simulink model "Model"  (R2023b)
settings: Solver=VariableStepAuto  StartTime=0.0  StopTime=10.0  RelTol=1e-3
values from neighbouring files (symbols this model uses):
  sys = System()    [Aflevering_3.m]
libraries: slpidlib x4
settings Model: Creator=JesperBertelsen  LastModifiedBy=JesperBertelsen

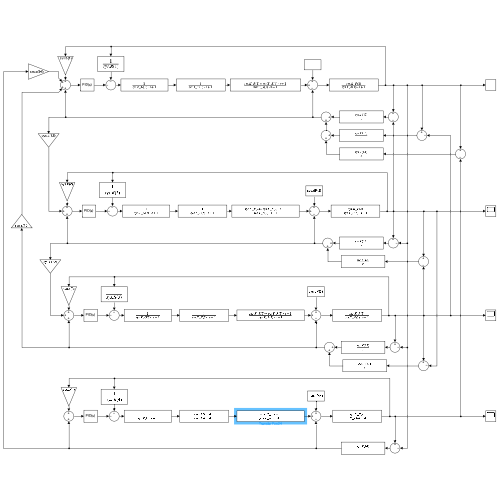
[thumbnail: Simulink's stored preview of the top-level diagram]
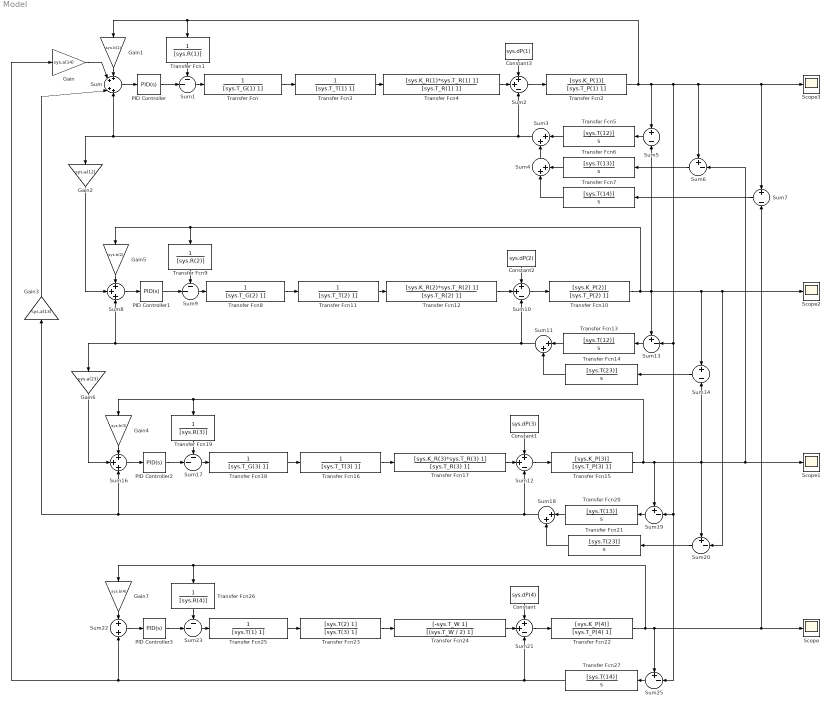
== system Model ==
  Constant : Constant  Value=sys.dP(4)
  Constant1 : Constant  Value=sys.dP(3)
  Constant2 : Constant  Value=sys.dP(2)
  Constant3 : Constant  Value=sys.dP(1)
  Gain : Gain  Gain=sys.a(14)
  Gain1 : Gain  Gain=sys.b(1)
  Gain2 : Gain  Gain=sys.a(12)
  Gain3 : Gain  Gain=sys.a(13)
  Gain4 : Gain  Gain=sys.b(3)
  Gain5 : Gain  Gain=sys.b(2)
  Gain6 : Gain  Gain=sys.a(23)
  Gain7 : Gain  Gain=sys.b(4)
  PID Controller{,1..3} (4 alike) : slpidlib/PID Controller  Controller=PID  Form=Parallel  TimeDomain=Continuous-time  UseExternalTs=off  SampleTime=-1  IntegratorMethod=Forward Euler  FilterMethod=Forward Euler  ControllerParametersSource=internal  P=1  I=1  UseKiTs=off  D=0  N=100  UseFilter=on  TunerSelectOption=Transfer Function Based (PID Tuner App)  InitialConditionSource=internal  InitialConditionForIntegrator=0  InitialConditionForFilter=0  DifferentiatorICPrevScaledInput=0  ExternalReset=none  TrackingMode=off  Kt=1  LimitOutput=off  SatLimitsSource=internal  UpperSaturationLimit=inf  LowerSaturationLimit=-inf  LinearizeAsGain=on  AntiWindupMode=none  Kb=1  LimitIntegrator=off  UpperIntegratorSaturationLimit=inf  LowerIntegratorSaturationLimit=-inf  POutMin=[]  POutMax=[]  IOutMin=[]  IOutMax=[]  DOutMin=[]  DOutMax=[]  NOutMin=[]  NOutMax=[]  SumOutMin=[]  SumOutMax=[]  SaturationOutMin=[]  SaturationOutMax=[]  PParamMin=[]  PParamMax=[]  IParamMin=[]  IParamMax=[]  DParamMin=[]  DParamMax=[]  NParamMin=[]  NParamMax=[]  KbParamMin=[]  KbParamMax=[]  KtParamMin=[]  KtParamMax=[]  KbOutMin=[]  KbOutMax=[]  KtOutMin=[]  KtOutMax=[]  IntegratorOutMin=[]  IntegratorOutMax=[]  FilterOutMin=[]  FilterOutMax=[]  SumI1OutMin=[]  SumI1OutMax=[]  SumI2OutMin=[]  SumI2OutMax=[]  SumI3OutMin=[]  SumI3OutMax=[]  SumI4OutMin=[]  SumI4OutMax=[]  SumDOutMin=[]  SumDOutMax=[]  DifferentiatorOutMin=[]  DifferentiatorOutMax=[]  FilterDiffOutCoefMin=[]  FilterDiffOutCoefMax=[]  ReciprocalOutMin=[]  ReciprocalOutMax=[]  SumDenOutMin=[]  SumDenOutMax=[]  SumNumOutMin=[]  SumNumOutMax=[]  DivideOutMin=[]  DivideOutMax=[]  UdiffTsProdOutMin=[]  UdiffTsProdOutMax=[]  NTsProdOutMin=[]  NTsProdOutMax=[]  UintegralTsProdOutMin=[]  UintegralTsProdOutMax=[]  UngainTsProdOutMin=[]  UngainTsProdOutMax=[]  ClampingZeroOutDataTypeStr=Inherit: Inherit via back propagation  ClampingZeroOutMin=[]  ClampingZeroOutMax=[]  FilterDenConstantOutDataTypeStr=Inherit: Inherit via back propagation  FilterDenConstantOutMin=[]  FilterDenConstantOutMax=[]  PCopyOutDataTypeStr=Inherit: Inherit via back propagation  PCopyOutMin=[]  PCopyOutMax=[]  NCopyOutDataTypeStr=Inherit: Inherit via back propagation  NCopyOutMin=[]  NCopyOutMax=[]  IntegratorContinuousStateAttributes=''  IntegratorStateMustResolveToSignalObject=off  IntegratorRTWStateStorageClass=Auto  FilterContinuousStateAttributes=''  FilterStateMustResolveToSignalObject=off  FilterRTWStateStorageClass=Auto  ParallelPVariant=InternalParameters  IdealPVariant=Disabled  IVariant=InternalParameters  DVariant=InternalParameters  IntegratorVariant=Continuous  SatVariant=Disabled  AWVariant=Passthrough  PCopyVariant=Disabled  TRVariant=Disabled  FdbkBlocksVariant=Forward  IdealPFdbkVariant=Disabled  SatFdbkVariant=Disabled  DerivativeFilterVariant=ContFilter  NVariant=InternalParameters  NCopyVariant=Disabled  FilterICVariant=InternalICsFilter  IntegratorICVariant=InternalICs  ExternalResetVariant=Disabled  TRSumVariant=Passthrough  SumFdbkVariant=Disabled  SumVariant=Sum_PID  TsampFilterVariant=InternalTs  TsampNgainVariant=Passthrough  TsampIntegralVariant=Disabled_SignalSpec  ExternalSaturationOutDataTypeStr=Inherit: Same as second input
  Scope{,1..3} (4 alike) : Scope
  Sum : Sum  Inputs=++|++
  Sum{1,9,17,23} (4 alike) : Sum  Inputs=--|
  Sum{2,10,12,21} (4 alike) : Sum  Inputs=++-
  Sum{3..4,11,18} (4 alike) : Sum  Inputs=|++
  Sum{6,13,19..20,25} (5 alike) : Sum  Inputs=+-|
  Sum14 : Sum  Inputs=+-
  Sum16 : Sum  Inputs=+++
  Sum22 : Sum  Inputs=+|+
  Sum5 : Sum  Inputs=+|-
  Sum7 : Sum  Inputs=+|-
  Sum8 : Sum  Inputs=+++
  Transfer Fcn : TransferFcn  Denominator=[sys.T_G(1) 1]
  Transfer Fcn1 : TransferFcn  Denominator=[sys.R(1)]
  Transfer Fcn10 : TransferFcn  Numerator=[sys.K_P(2)]  Denominator=[sys.T_P(2) 1]
  Transfer Fcn11 : TransferFcn  Denominator=[sys.T_T(2) 1]
  Transfer Fcn12 : TransferFcn  Numerator=[sys.K_R(2)*sys.T_R(2) 1]  Denominator=[sys.T_R(2) 1]
  Transfer Fcn13 : TransferFcn  Numerator=[sys.T(12)]  Denominator=[1 0]
  Transfer Fcn14 : TransferFcn  Numerator=[sys.T(23)]  Denominator=[1 0]
  Transfer Fcn15 : TransferFcn  Numerator=[sys.K_P(3)]  Denominator=[sys.T_P(3) 1]
  Transfer Fcn16 : TransferFcn  Denominator=[sys.T_T(3) 1]
  Transfer Fcn17 : TransferFcn  Numerator=[sys.K_R(3)*sys.T_R(3) 1]  Denominator=[sys.T_R(3) 1]
  Transfer Fcn18 : TransferFcn  Denominator=[sys.T_G(3) 1]
  Transfer Fcn19 : TransferFcn  Denominator=[sys.R(3)]
  Transfer Fcn2 : TransferFcn  Numerator=[sys.K_P(1)]  Denominator=[sys.T_P(1) 1]
  Transfer Fcn20 : TransferFcn  Numerator=[sys.T(13)]  Denominator=[1 0]
  Transfer Fcn21 : TransferFcn  Numerator=[sys.T(23)]  Denominator=[1 0]
  Transfer Fcn22 : TransferFcn  Numerator=[sys.K_P(4)]  Denominator=[sys.T_P(4) 1]
  Transfer Fcn23 : TransferFcn  Numerator=[sys.T(2) 1]  Denominator=[sys.T(3) 1]
  Transfer Fcn24 : TransferFcn  Numerator=[-sys.T_W 1]  Denominator=[(sys.T_W / 2) 1]
  Transfer Fcn25 : TransferFcn  Denominator=[sys.T(1) 1]
  Transfer Fcn26 : TransferFcn  Denominator=[sys.R(4)]
  Transfer Fcn27 : TransferFcn  Numerator=[sys.T(14)]  Denominator=[1 0]
  Transfer Fcn3 : TransferFcn  Denominator=[sys.T_T(1) 1]
  Transfer Fcn4 : TransferFcn  Numerator=[sys.K_R(1)*sys.T_R(1) 1]  Denominator=[sys.T_R(1) 1]
  Transfer Fcn5 : TransferFcn  Numerator=[sys.T(12)]  Denominator=[1 0]
  Transfer Fcn6 : TransferFcn  Numerator=[sys.T(13)]  Denominator=[1 0]
  Transfer Fcn7 : TransferFcn  Numerator=[sys.T(14)]  Denominator=[1 0]
  Transfer Fcn8 : TransferFcn  Denominator=[sys.T_G(2) 1]
  Transfer Fcn9 : TransferFcn  Denominator=[sys.R(2)]
  wires:
  Sum/1 -> PID Controller/1
  Transfer Fcn/1 -> Transfer Fcn3/1
  Sum1/1 -> Transfer Fcn/1
  Transfer Fcn4/1 -> Sum2/2
  Transfer Fcn3/1 -> Transfer Fcn4/1
  Transfer Fcn2/1 -> Sum5/1, Sum13/2, Sum19/2, Sum25/2, Sum6/1, Sum7/1, Scope3/1, Transfer Fcn1/1, Gain1/1
  Sum2/1 -> Transfer Fcn2/1
  PID Controller/1 -> Sum1/2
  Transfer Fcn1/1 -> Sum1/1
  Gain/1 -> Sum/2
  Gain1/1 -> Sum/1
  Sum3/1 -> Sum2/3, Gain2/1, Sum/4
  Transfer Fcn5/1 -> Sum3/1
  Transfer Fcn6/1 -> Sum4/2
  Sum4/1 -> Sum3/2
  Transfer Fcn7/1 -> Sum4/1
  Sum5/1 -> Transfer Fcn5/1
  Sum6/1 -> Transfer Fcn6/1
  Sum7/1 -> Transfer Fcn7/1
  Gain3/1 -> Sum/3
  Transfer Fcn8/1 -> Transfer Fcn11/1
  Gain5/1 -> Sum8/1
  Transfer Fcn11/1 -> Transfer Fcn12/1
  Sum10/1 -> Transfer Fcn10/1
  PID Controller1/1 -> Sum9/2
  Gain2/1 -> Sum8/2
  Transfer Fcn10/1 -> Sum13/1, Sum5/2, Sum14/1, Scope2/1, Sum20/2, Transfer Fcn9/1, Gain5/1
  Transfer Fcn9/1 -> Sum9/1
  Sum9/1 -> Transfer Fcn8/1
  Sum8/1 -> PID Controller1/1
  Sum11/1 -> Sum10/3, Sum8/3, Gain6/1
  Transfer Fcn12/1 -> Sum10/2
  Sum14/1 -> Transfer Fcn14/1
  Transfer Fcn13/1 -> Sum11/1
  Sum13/1 -> Transfer Fcn13/1
  Transfer Fcn14/1 -> Sum11/2
  Transfer Fcn18/1 -> Transfer Fcn16/1
  Transfer Fcn17/1 -> Sum12/2
  Sum17/1 -> Transfer Fcn18/1
  PID Controller2/1 -> Sum17/2
  Gain4/1 -> Sum16/1
  Transfer Fcn16/1 -> Transfer Fcn17/1
  Sum16/1 -> PID Controller2/1
  Sum12/1 -> Transfer Fcn15/1
  Transfer Fcn19/1 -> Sum17/1
  Gain6/1 -> Sum16/2
  Sum20/1 -> Transfer Fcn21/1
  Transfer Fcn21/1 -> Sum18/2
  Transfer Fcn20/1 -> Sum18/1
  Sum19/1 -> Transfer Fcn20/1
  Transfer Fcn15/1 -> Sum6/2, Scope1/1, Sum14/2, Sum20/1, Sum19/1, Transfer Fcn19/1, Gain4/1
  Sum18/1 -> Gain3/1, Sum16/3, Sum12/3
  Sum21/1 -> Transfer Fcn22/1
  Sum25/1 -> Transfer Fcn27/1
  Gain7/1 -> Sum22/1
  Transfer Fcn25/1 -> Transfer Fcn23/1
  Transfer Fcn24/1 -> Sum21/2
  Sum23/1 -> Transfer Fcn25/1
  Transfer Fcn23/1 -> Transfer Fcn24/1
  PID Controller3/1 -> Sum23/2
  Sum22/1 -> PID Controller3/1
  Transfer Fcn22/1 -> Transfer Fcn26/1, Gain7/1, Scope/1, Sum7/2, Sum25/1
  Transfer Fcn26/1 -> Sum23/1
  Transfer Fcn27/1 -> Gain/1, Sum22/2, Sum21/3
  Constant/1 -> Sum21/1
  Constant1/1 -> Sum12/1
  Constant2/1 -> Sum10/1
  Constant3/1 -> Sum2/1
